simulink model "scotch_yoke_model"  (R2024b)
settings: Solver=VariableStepAuto  StartTime=0.0  StopTime=10  RelTol=1e-3
values from neighbouring files (symbols this model uses):
  c_linear = 5000    [model_params.m]
  I_disk = (1/2)* M_disk * (disk_diameter/2)^2    (= 0.000725807903229)    [model_params.m]
  M_cart = 0.5    [model_params.m]
  R_crank = 1 / 39.37    (= 0.0254000508001)    [model_params.m]
  theta0 = 0    [model_params.m]
  theta0_dot = 0    [model_params.m]
settings Model: Creator=lucas  LastModifiedBy=lucas

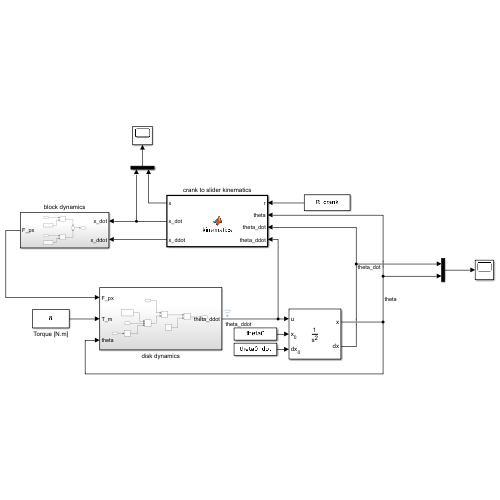
[thumbnail: Simulink's stored preview of the top-level diagram]
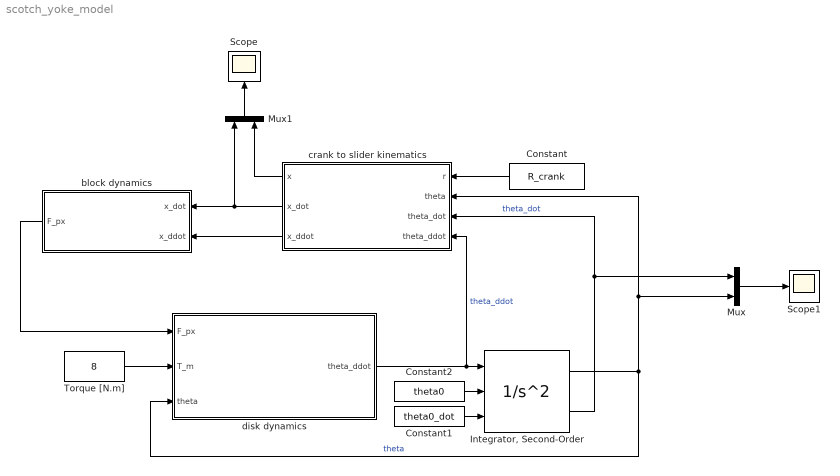
== system scotch_yoke_model ==
  Constant : Constant  Value=R_crank
  Constant1 : Constant  Value=theta0_dot
  Constant2 : Constant  Value=theta0
  "Integrator, Second-Order" : SecondOrderIntegrator  ICSourceX=external  ICSourceDXDT=external
  Mux : Mux  Inputs=2
  Mux1 : Mux  Inputs=2
  Scope : Scope
  Scope1 : Scope
  Torque [N.m] : Constant  Value=8
  block dynamics : Subsystem
  crank to slider kinematics : MATLAB Function  TreatAsAtomicUnit=on
  disk dynamics : Subsystem
  wires:
  Constant/1 -> crank to slider kinematics/1(r)
  crank to slider kinematics/2(x_dot) -> Mux1/1, block dynamics/1(x_dot)
  crank to slider kinematics/3(x_ddot) -> block dynamics/2(x_ddot)
  block dynamics/1(F_px) -> disk dynamics/1(F_px)
  Torque [N.m]/1 -> disk dynamics/2(T_m)
  "Integrator, Second-Order"/2 -> crank to slider kinematics/3(theta_dot), Mux/1  "theta_dot"
  disk dynamics/1(theta_ddot) -> crank to slider kinematics/4(theta_ddot), "Integrator, Second-Order"/1  "theta_ddot"
  "Integrator, Second-Order"/1 -> disk dynamics/3(theta), Mux/2, crank to slider kinematics/2(theta)  "theta"
  Constant2/1 -> "Integrator, Second-Order"/2
  Constant1/1 -> "Integrator, Second-Order"/3
  Mux/1 -> Scope1/1
  crank to slider kinematics/1(x) -> Mux1/2
  Mux1/1 -> Scope/1

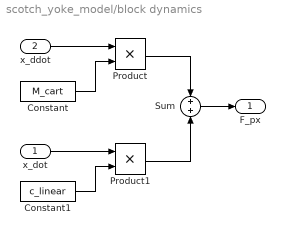
== system scotch_yoke_model/block dynamics ==
  x_dot : Inport
  x_ddot : Inport  Port=2
  Constant : Constant  Value=M_cart
  Constant1 : Constant  Value=c_linear
  Product : Product
  Product1 : Product
  Sum : Sum  Inputs=+|+
  F_px : Outport
  wires:
  x_ddot/1 -> Product/1
  Constant/1 -> Product/2
  x_dot/1 -> Product1/1
  Constant1/1 -> Product1/2
  Product/1 -> Sum/1
  Product1/1 -> Sum/2
  Sum/1 -> F_px/1

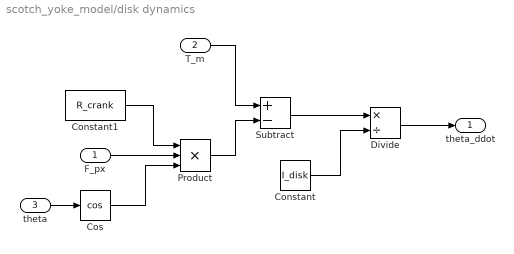
== system scotch_yoke_model/disk dynamics ==
  F_px : Inport
  T_m : Inport  Port=2
  theta : Inport  Port=3
  Constant : Constant  Value=I_disk
  Constant1 : Constant  Value=R_crank
  Cos : Trigonometry  Operator=cos
  Divide : Product  Inputs=*/
  Product : Product  Inputs=3
  Subtract : Sum  Inputs=+-
  theta_ddot : Outport
  wires:
  Constant/1 -> Divide/2
  theta/1 -> Cos/1
  Constant1/1 -> Product/1
  F_px/1 -> Product/2
  Cos/1 -> Product/3
  Product/1 -> Subtract/2
  T_m/1 -> Subtract/1
  Subtract/1 -> Divide/1
  Divide/1 -> theta_ddot/1

== matlab function scotch_yoke_model/crank to slider kinematics ==
  data: r input; x output; theta input; theta_dot input; theta_ddot input; x_dot output; x_ddot output
function [x, x_dot, x_ddot] = kinematics(r, theta, theta_dot, theta_ddot)

x = r * sin(theta);
x_dot = r * theta_dot*cos(theta);
x_ddot = r*(theta_ddot * cos(theta) - theta_dot^2 * sin(theta));

end
